simulink model "IMU_Uno"  (R2025b)
settings: Solver=FixedStepAuto  StartTime=0.0  StopTime=inf  FixedStep=Ts  RelTol=1e-3  EnableMultiTasking=on
InitFcn:
  | Ts=0.01;
  | Delay=5;
  | Av=50;
  | Sample_div=uint8(9);
  | Filter_BW=uint8(5);  %bandwidth 10 Hz
  | Gy_Conf=uint8(24); %-2000dps to 2000dps
  | Acc_Conf1=uint8(0); % -2g to 2g
  | Acc_Conf2=uint8(5); % bandwidth 10 Hz
  | FIFO_en=uint8(0); % Disabled
  | INT_en=uint8(0); % Disabled
  | Acc_Scale=9.8*2/32767;
  | Gyro_Scale=(2000*pi/180)/32767;
  | g_offset=16384;
  | 
  | %Registers
  | IMU_ID=113;
  | IMU_Add=104;
  | Who_Am_I=117;
  | PWR_1=107;
  | PWR_2=108;
  | SAMPL_DIV=25;
  | CONFIG_REG=26;
  | GYRO_CONFIG=27;
  | ACC_CONFIG_1=28;
  | ACC_CONFIG_2=29;
  | FIFO_EN=35;
  | INT_EN=56;
  | GY_X_OFFSET_H=19;
  | GY_X_OFFSET_L=20;
  | GY_Y_OFFSET_H=21;
  | GY_Y_OFFSET_L=22;
  | GY_Z_OFFSET_H=23;
  | GY_Z_OFFSET_L=24;
  | ACC_X_OFFSET_H=119;
  | ACC_X_OFFSET_L=120;
  | ACC_Y_OFFSET_H=122;
  | ACC_Y_OFFSET_L=123;
  | ACC_Z_OFFSET_H=125;
  | ACC_Z_OFFSET_L=126;
  | ACCEL_XOUT_H=59;
  | ACCEL_XOUT_L=60;
  | ACCEL_YOUT_H=61;
  | ACCEL_YOUT_L=62;
  | ACCEL_ZOUT_H=63;
  | ACCEL_ZOUT_L=64;
  | GYRO_XOUT_H=67;
  | GYRO_XOUT_L=68;
  | GYRO_YOUT_H=69;
  | GYRO_YOUT_L=70;
  | GYRO_ZOUT_H=71;
  | GYRO_ZOUT_L=72;
libraries: arduinolib x18
settings Model: SimulationMode=external  ExtModeTrigDuration=2  Creator=amind  LastModifiedBy=Amin Danial
settings SolverCC: AlgebraicLoopSolver=TrustRegion  AutoInsertRateTranBlk=on
settings DataIOCC: ReturnWorkspaceOutputs=off
settings OptimizationCC: EnhancedBackFolding=on  PassReuseOutputArgsAs=Individual arguments  MaxStackSize=64  OptimizeBlockOrder=speed  DifferentSizesBufferReuse=on  OptimizationCustomize=off  EfficientTunableParamExpr=on
settings DebuggingCC: ParameterPrecisionLossMsg=none  ParameterTunabilityLossMsg=error  UnconnectedInputMsg=warning  UnconnectedOutputMsg=warning  UnconnectedLineMsg=warning  ArithmeticOperatorsInVariantConditions=warning
settings HardwareCC: ProdBitPerInt=16.0  ProdBitPerPointer=16.0  ProdBitPerSizeT=16.0  ProdBitPerPtrDiffT=16.0  ProdLargestAtomicFloat=None  ProdWordSize=8.0  ProdHWDeviceType=Atmel->AVR
settings ModelReferenceCC: EnableRefExpFcnMdlSchedulingChecks=on
settings SFSimCC: MATLABDynamicMemAlloc=off  CustomCodeUndefinedFunction=UseInterfaceOnly
settings RTWCC: SystemTargetFile=ert.tlc  HardwareBoard=Arduino Uno  TemplateMakefile=ert_default_tmf  GenerateReport=on  Toolchain=Arduino AVR  BuildConfiguration=Faster Runs  IncludeHyperlinkInReport=on  LaunchReport=on  GenerateTraceInfo=on  GenerateTraceReport=on  GenerateTraceReportSl=on  GenerateTraceReportSf=on  GenerateTraceReportEml=on  GPUComputeCapability=3.5  Description=Embedded Coder
settings CodeAppCC: ForceParamTrailComments=on  IgnoreCustomStorageClasses=off  OperatorAnnotations=on  SimulinkDataObjDesc=on  SFDataObjDesc=on  InsertBlockDesc=on
settings ERTTargetCC: ExtModeTransport=3.0  ExtModeStaticAlloc=on  ExtModeAutomaticAllocSize=off  ExtModeStaticAllocSize=250.0  ExtModeMexFile=ext_xcp  ExtModeIntrfLevel=Level2 - Open  InlinedParameterPlacement=Hierarchical  DynamicArrayContainerType=coder::array  SupportContinuousTime=on  SupportVariableSizeSignals=on

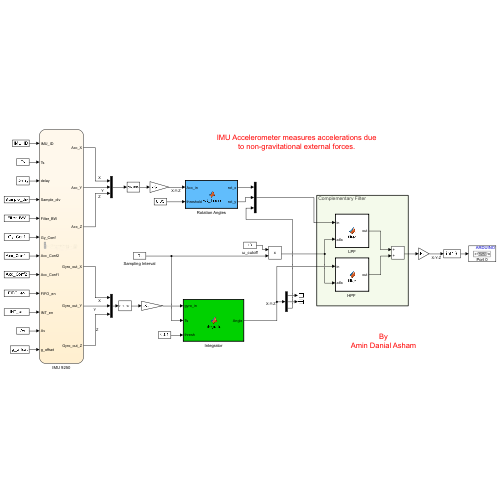
[thumbnail: Simulink's stored preview of the top-level diagram]
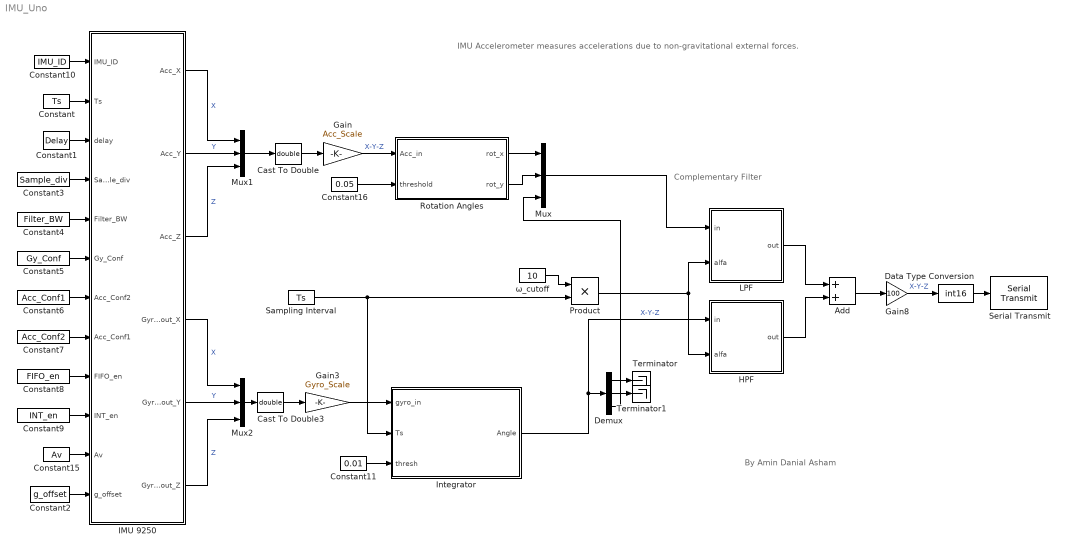
== system IMU_Uno ==
  note: By
      | Amin Danial Asham
  note: IMU Accelerometer measures accelerations due to non-gravitational external forces.
  note: Complementary Filter
  Add : Sum
  Cast To Double : DataTypeConversion  OutDataTypeStr=double  SaturateOnIntegerOverflow=off  RndMeth=Floor
  Cast To Double3 : DataTypeConversion  OutDataTypeStr=double  SaturateOnIntegerOverflow=off  RndMeth=Floor
  Constant : Constant  Value=Ts
  Constant1 : Constant  Value=Delay
  Constant10 : Constant  Value=IMU_ID
  Constant11 : Constant  Value=0.01
  Constant15 : Constant  Value=Av
  Constant16 : Constant  Value=0.05
  Constant2 : Constant  Value=g_offset
  Constant3 : Constant  Value=Sample_div
  Constant4 : Constant  Value=Filter_BW
  Constant5 : Constant  Value=Gy_Conf
  Constant6 : Constant  Value=Acc_Conf1
  Constant7 : Constant  Value=Acc_Conf2
  Constant8 : Constant  Value=FIFO_en
  Constant9 : Constant  Value=INT_en
  Data Type Conversion : DataTypeConversion  OutDataTypeStr=int16  SaturateOnIntegerOverflow=off  RndMeth=Floor
  Demux : Demux  Outputs=3
  Gain : Gain  Gain=Acc_Scale
  Gain3 : Gain  Gain=Gyro_Scale
  Gain8 : Gain  Gain=100
  "HPF " : MATLAB Function  TreatAsAtomicUnit=on
  IMU 9250 : Stateflow chart  TreatAsAtomicUnit=on  SystemSampleTime=Ts
  Integrator : MATLAB Function  InitFcn=|  TreatAsAtomicUnit=on
      | gyro=zeros(3,1);
      | gyro_1=zeros(3,1);
      | Angles=zeros(3,1);
  LPF : MATLAB Function  TreatAsAtomicUnit=on
  Mux : Mux  Inputs=3
  Mux1 : Mux  Inputs=3
  Mux2 : Mux  Inputs=3
  Product : Product
  Rotation Angles : MATLAB Function  TreatAsAtomicUnit=on
  Sampling Interval : Constant  Value=Ts
  Serial Transmit : arduinolib/Serial Transmit  portNumber=0  sendmode=write  sendformat=Decimal  floatprecision=2  header=[]  terminator=[]  blockPlatform=arduino
  Terminator : Terminator
  Terminator1 : Terminator
  ω_cutoff : Constant  Value=10
  wires:
  IMU 9250/1(Acc_X) -> Mux1/1  "X"
  IMU 9250/3(Acc_Z) -> Mux1/3  "Z"
  IMU 9250/2(Acc_Y) -> Mux1/2  "Y"
  Rotation Angles/1(rot_x) -> Mux/1
  Rotation Angles/2(rot_y) -> Mux/2
  Mux2/1 -> Cast To Double3/1
  IMU 9250/4(Gyro_out_X) -> Mux2/1  "X"
  IMU 9250/5(Gyro_out_Y) -> Mux2/2  "Y"
  IMU 9250/6(Gyro_out_Z) -> Mux2/3  "Z"
  Cast To Double3/1 -> Gain3/1
  Mux/1 -> LPF/1(in)
  Gain8/1 -> Data Type Conversion/1  "X-Y-Z"
  Data Type Conversion/1 -> Serial Transmit/1
  LPF/1(out) -> Add/1
  Mux1/1 -> Cast To Double/1
  Constant2/1 -> IMU 9250/12(g_offset)
  Constant15/1 -> IMU 9250/11(Av)
  Constant10/1 -> IMU 9250/1(IMU_ID)
  Constant6/1 -> IMU 9250/7(Acc_Conf2)
  Constant3/1 -> IMU 9250/4(Sample_div)
  Constant4/1 -> IMU 9250/5(Filter_BW)
  Constant5/1 -> IMU 9250/6(Gy_Conf)
  Constant9/1 -> IMU 9250/10(INT_en)
  Constant1/1 -> IMU 9250/3(delay)
  Constant7/1 -> IMU 9250/8(Acc_Conf1)
  Constant/1 -> IMU 9250/2(Ts)
  Constant8/1 -> IMU 9250/9(FIFO_en)
  Constant16/1 -> Rotation Angles/2(threshold)
  Cast To Double/1 -> Gain/1
  Gain/1 -> Rotation Angles/1(Acc_in)  "X-Y-Z"
  Product/1 -> LPF/2(alfa), "HPF "/2(alfa)
  Integrator/1(Angle) -> "HPF "/1(in), Demux/1  "X-Y-Z"
  Demux/3 -> Mux/3
  Demux/1 -> Terminator/1
  Demux/2 -> Terminator1/1
  "HPF "/1(out) -> Add/2
  Add/1 -> Gain8/1
  Sampling Interval/1 -> Integrator/2(Ts), Product/2
  ω_cutoff/1 -> Product/1
  Gain3/1 -> Integrator/1(gyro_in)
  Constant11/1 -> Integrator/3(thresh)

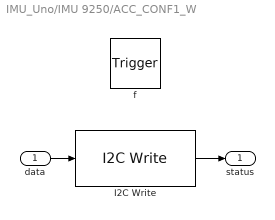
== system IMU_Uno/IMU 9250/ACC_CONF1_W ==
  data : Inport  OutDataTypeStr=uint8  PortDimensions=1
  f : TriggerPort  TriggerType=function-call  VariantControl=(inherit)
      settings: CopyFcn=Stateflow.SLINSF.SimulinkMan.removeBlockPreDeleteFcn  PreDeleteFcn=Stateflow.SLINSF.SimulinkMan.unsafePredeleteFcn
  I2C Write : arduinolib/I2C Write  I2CModule=0  Mode=Master  SlaveAddress=IMU_Add  SlaveByteOrder=BigEndian  Direction=Transmitter  RegisterAddressMode=on  RegisterAddress=ACC_CONFIG_1  SlaveDataType=uint8  DataLength=1  NoAck=off  RepeatedStart=off  OutputStatus=on  blockPlatform=ARDUINO
  status : Outport  VectorParamsAs1DForOutWhenUnconnected=off
  wires:
  I2C Write/1 -> status/1
  data/1 -> I2C Write/1

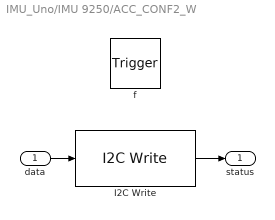
== system IMU_Uno/IMU 9250/ACC_CONF2_W ==
  data : Inport  OutDataTypeStr=uint8  PortDimensions=1
  f : TriggerPort  TriggerType=function-call  VariantControl=(inherit)
      settings: CopyFcn=Stateflow.SLINSF.SimulinkMan.removeBlockPreDeleteFcn  PreDeleteFcn=Stateflow.SLINSF.SimulinkMan.unsafePredeleteFcn
  I2C Write : arduinolib/I2C Write  I2CModule=0  Mode=Master  SlaveAddress=IMU_Add  SlaveByteOrder=BigEndian  Direction=Transmitter  RegisterAddressMode=on  RegisterAddress=ACC_CONFIG_2  SlaveDataType=uint8  DataLength=1  NoAck=off  RepeatedStart=off  OutputStatus=on  blockPlatform=ARDUINO
  status : Outport  VectorParamsAs1DForOutWhenUnconnected=off
  wires:
  I2C Write/1 -> status/1
  data/1 -> I2C Write/1

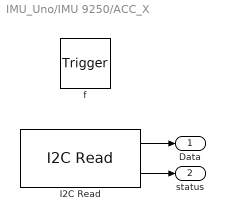
== system IMU_Uno/IMU 9250/ACC_X ==
  f : TriggerPort  TriggerType=function-call  VariantControl=(inherit)
      settings: CopyFcn=Stateflow.SLINSF.SimulinkMan.removeBlockPreDeleteFcn  PreDeleteFcn=Stateflow.SLINSF.SimulinkMan.unsafePredeleteFcn
  I2C Read : arduinolib/I2C Read  I2CModule=0  Mode=Master  SlaveAddress=IMU_Add  SlaveByteOrder=BigEndian  Direction=Receiver  RegisterAddressMode=on  RegisterAddress=ACCEL_XOUT_H  SlaveDataType=int16  DataLength=1  NoAck=off  RepeatedStart=off  OutputStatus=on  blockPlatform=ARDUINO  SampleTime=-1
  Data : Outport  VectorParamsAs1DForOutWhenUnconnected=off
  status : Outport  Port=2  VectorParamsAs1DForOutWhenUnconnected=off
  wires:
  I2C Read/1 -> Data/1
  I2C Read/2 -> status/1

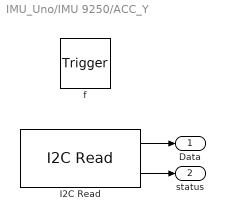
== system IMU_Uno/IMU 9250/ACC_Y ==
  f : TriggerPort  TriggerType=function-call  VariantControl=(inherit)
      settings: CopyFcn=Stateflow.SLINSF.SimulinkMan.removeBlockPreDeleteFcn  PreDeleteFcn=Stateflow.SLINSF.SimulinkMan.unsafePredeleteFcn
  I2C Read : arduinolib/I2C Read  I2CModule=0  Mode=Master  SlaveAddress=IMU_Add  SlaveByteOrder=BigEndian  Direction=Receiver  RegisterAddressMode=on  RegisterAddress=ACCEL_YOUT_H  SlaveDataType=int16  DataLength=1  NoAck=off  RepeatedStart=off  OutputStatus=on  blockPlatform=ARDUINO  SampleTime=-1
  Data : Outport  VectorParamsAs1DForOutWhenUnconnected=off
  status : Outport  Port=2  VectorParamsAs1DForOutWhenUnconnected=off
  wires:
  I2C Read/1 -> Data/1
  I2C Read/2 -> status/1

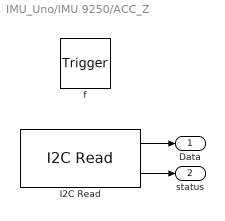
== system IMU_Uno/IMU 9250/ACC_Z ==
  f : TriggerPort  TriggerType=function-call  VariantControl=(inherit)
      settings: CopyFcn=Stateflow.SLINSF.SimulinkMan.removeBlockPreDeleteFcn  PreDeleteFcn=Stateflow.SLINSF.SimulinkMan.unsafePredeleteFcn
  I2C Read : arduinolib/I2C Read  I2CModule=0  Mode=Master  SlaveAddress=IMU_Add  SlaveByteOrder=BigEndian  Direction=Receiver  RegisterAddressMode=on  RegisterAddress=ACCEL_ZOUT_H  SlaveDataType=int16  DataLength=1  NoAck=off  RepeatedStart=off  OutputStatus=on  blockPlatform=ARDUINO  SampleTime=-1
  Data : Outport  VectorParamsAs1DForOutWhenUnconnected=off
  status : Outport  Port=2  VectorParamsAs1DForOutWhenUnconnected=off
  wires:
  I2C Read/1 -> Data/1
  I2C Read/2 -> status/1

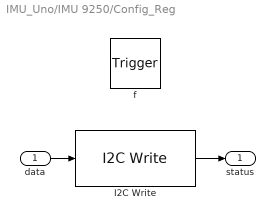
== system IMU_Uno/IMU 9250/Config_Reg ==
  data : Inport  OutDataTypeStr=uint8  PortDimensions=1
  f : TriggerPort  TriggerType=function-call  VariantControl=(inherit)
      settings: CopyFcn=Stateflow.SLINSF.SimulinkMan.removeBlockPreDeleteFcn  PreDeleteFcn=Stateflow.SLINSF.SimulinkMan.unsafePredeleteFcn
  I2C Write : arduinolib/I2C Write  I2CModule=0  Mode=Master  SlaveAddress=IMU_Add  SlaveByteOrder=BigEndian  Direction=Transmitter  RegisterAddressMode=on  RegisterAddress=CONFIG_REG  SlaveDataType=uint8  DataLength=1  NoAck=off  RepeatedStart=off  OutputStatus=on  blockPlatform=ARDUINO
  status : Outport  VectorParamsAs1DForOutWhenUnconnected=off
  wires:
  I2C Write/1 -> status/1
  data/1 -> I2C Write/1

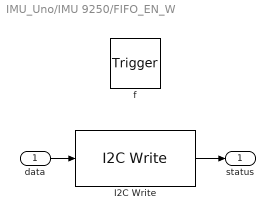
== system IMU_Uno/IMU 9250/FIFO_EN_W ==
  data : Inport  OutDataTypeStr=uint8  PortDimensions=1
  f : TriggerPort  TriggerType=function-call  VariantControl=(inherit)
      settings: CopyFcn=Stateflow.SLINSF.SimulinkMan.removeBlockPreDeleteFcn  PreDeleteFcn=Stateflow.SLINSF.SimulinkMan.unsafePredeleteFcn
  I2C Write : arduinolib/I2C Write  I2CModule=0  Mode=Master  SlaveAddress=IMU_Add  SlaveByteOrder=BigEndian  Direction=Transmitter  RegisterAddressMode=on  RegisterAddress=FIFO_EN  SlaveDataType=uint8  DataLength=1  NoAck=off  RepeatedStart=off  OutputStatus=on  blockPlatform=ARDUINO
  status : Outport  VectorParamsAs1DForOutWhenUnconnected=off
  wires:
  I2C Write/1 -> status/1
  data/1 -> I2C Write/1

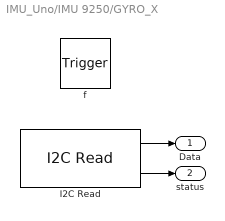
== system IMU_Uno/IMU 9250/GYRO_X ==
  f : TriggerPort  TriggerType=function-call  VariantControl=(inherit)
      settings: CopyFcn=Stateflow.SLINSF.SimulinkMan.removeBlockPreDeleteFcn  PreDeleteFcn=Stateflow.SLINSF.SimulinkMan.unsafePredeleteFcn
  I2C Read : arduinolib/I2C Read  I2CModule=0  Mode=Master  SlaveAddress=IMU_Add  SlaveByteOrder=BigEndian  Direction=Receiver  RegisterAddressMode=on  RegisterAddress=GYRO_XOUT_H  SlaveDataType=int16  DataLength=1  NoAck=off  RepeatedStart=off  OutputStatus=on  blockPlatform=ARDUINO  SampleTime=-1
  Data : Outport  VectorParamsAs1DForOutWhenUnconnected=off
  status : Outport  Port=2  VectorParamsAs1DForOutWhenUnconnected=off
  wires:
  I2C Read/1 -> Data/1
  I2C Read/2 -> status/1

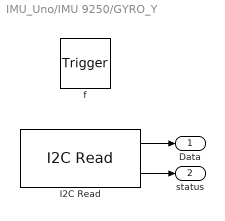
== system IMU_Uno/IMU 9250/GYRO_Y ==
  f : TriggerPort  TriggerType=function-call  VariantControl=(inherit)
      settings: CopyFcn=Stateflow.SLINSF.SimulinkMan.removeBlockPreDeleteFcn  PreDeleteFcn=Stateflow.SLINSF.SimulinkMan.unsafePredeleteFcn
  I2C Read : arduinolib/I2C Read  I2CModule=0  Mode=Master  SlaveAddress=IMU_Add  SlaveByteOrder=BigEndian  Direction=Receiver  RegisterAddressMode=on  RegisterAddress=GYRO_YOUT_H  SlaveDataType=int16  DataLength=1  NoAck=off  RepeatedStart=off  OutputStatus=on  blockPlatform=ARDUINO  SampleTime=-1
  Data : Outport  VectorParamsAs1DForOutWhenUnconnected=off
  status : Outport  Port=2  VectorParamsAs1DForOutWhenUnconnected=off
  wires:
  I2C Read/1 -> Data/1
  I2C Read/2 -> status/1

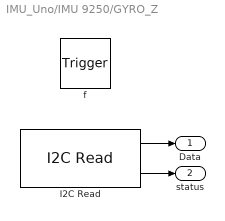
== system IMU_Uno/IMU 9250/GYRO_Z ==
  f : TriggerPort  TriggerType=function-call  VariantControl=(inherit)
      settings: CopyFcn=Stateflow.SLINSF.SimulinkMan.removeBlockPreDeleteFcn  PreDeleteFcn=Stateflow.SLINSF.SimulinkMan.unsafePredeleteFcn
  I2C Read : arduinolib/I2C Read  I2CModule=0  Mode=Master  SlaveAddress=IMU_Add  SlaveByteOrder=BigEndian  Direction=Receiver  RegisterAddressMode=on  RegisterAddress=GYRO_ZOUT_H  SlaveDataType=int16  DataLength=1  NoAck=off  RepeatedStart=off  OutputStatus=on  blockPlatform=ARDUINO  SampleTime=-1
  Data : Outport  VectorParamsAs1DForOutWhenUnconnected=off
  status : Outport  Port=2  VectorParamsAs1DForOutWhenUnconnected=off
  wires:
  I2C Read/1 -> Data/1
  I2C Read/2 -> status/1

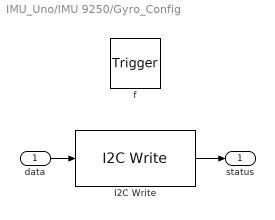
== system IMU_Uno/IMU 9250/Gyro_Config ==
  data : Inport  OutDataTypeStr=uint8  PortDimensions=1
  f : TriggerPort  TriggerType=function-call  VariantControl=(inherit)
      settings: CopyFcn=Stateflow.SLINSF.SimulinkMan.removeBlockPreDeleteFcn  PreDeleteFcn=Stateflow.SLINSF.SimulinkMan.unsafePredeleteFcn
  I2C Write : arduinolib/I2C Write  I2CModule=0  Mode=Master  SlaveAddress=IMU_Add  SlaveByteOrder=BigEndian  Direction=Transmitter  RegisterAddressMode=on  RegisterAddress=GYRO_CONFIG  SlaveDataType=uint8  DataLength=1  NoAck=off  RepeatedStart=off  OutputStatus=on  blockPlatform=ARDUINO
  status : Outport  VectorParamsAs1DForOutWhenUnconnected=off
  wires:
  I2C Write/1 -> status/1
  data/1 -> I2C Write/1

== system IMU_Uno/IMU 9250/INT_EN_W ==
  data : Inport  OutDataTypeStr=uint8  PortDimensions=1
  f : TriggerPort  TriggerType=function-call  VariantControl=(inherit)
      settings: CopyFcn=Stateflow.SLINSF.SimulinkMan.removeBlockPreDeleteFcn  PreDeleteFcn=Stateflow.SLINSF.SimulinkMan.unsafePredeleteFcn
  I2C Write : arduinolib/I2C Write  I2CModule=0  Mode=Master  SlaveAddress=IMU_Add  SlaveByteOrder=BigEndian  Direction=Transmitter  RegisterAddressMode=on  RegisterAddress=INT_EN  SlaveDataType=uint8  DataLength=1  NoAck=off  RepeatedStart=off  OutputStatus=on  blockPlatform=ARDUINO
  status : Outport  VectorParamsAs1DForOutWhenUnconnected=off
  wires:
  I2C Write/1 -> status/1
  data/1 -> I2C Write/1

== system IMU_Uno/IMU 9250/PWR1_R ==
  f : TriggerPort  TriggerType=function-call  VariantControl=(inherit)
      settings: CopyFcn=Stateflow.SLINSF.SimulinkMan.removeBlockPreDeleteFcn  PreDeleteFcn=Stateflow.SLINSF.SimulinkMan.unsafePredeleteFcn
  PWR 1 : arduinolib/I2C Read  I2CModule=0  Mode=Master  SlaveAddress=IMU_Add  SlaveByteOrder=BigEndian  Direction=Receiver  RegisterAddressMode=on  RegisterAddress=PWR_1  SlaveDataType=uint8  DataLength=1  NoAck=off  RepeatedStart=off  OutputStatus=on  blockPlatform=ARDUINO  SampleTime=-1
  data : Outport  VectorParamsAs1DForOutWhenUnconnected=off
  status : Outport  Port=2  VectorParamsAs1DForOutWhenUnconnected=off
  wires:
  PWR 1/1 -> data/1
  PWR 1/2 -> status/1

== system IMU_Uno/IMU 9250/PWR1_W ==
  data : Inport  OutDataTypeStr=uint8  PortDimensions=1
  f : TriggerPort  TriggerType=function-call  VariantControl=(inherit)
      settings: CopyFcn=Stateflow.SLINSF.SimulinkMan.removeBlockPreDeleteFcn  PreDeleteFcn=Stateflow.SLINSF.SimulinkMan.unsafePredeleteFcn
  PWR 1 1 : arduinolib/I2C Write  I2CModule=0  Mode=Master  SlaveAddress=IMU_Add  SlaveByteOrder=BigEndian  Direction=Transmitter  RegisterAddressMode=on  RegisterAddress=PWR_1  SlaveDataType=uint8  DataLength=1  NoAck=off  RepeatedStart=off  OutputStatus=on  blockPlatform=ARDUINO
  status : Outport  VectorParamsAs1DForOutWhenUnconnected=off
  wires:
  data/1 -> PWR 1 1/1
  PWR 1 1/1 -> status/1

== system IMU_Uno/IMU 9250/PWR2_W ==
  data : Inport  OutDataTypeStr=uint8  PortDimensions=1
  f : TriggerPort  TriggerType=function-call  VariantControl=(inherit)
      settings: CopyFcn=Stateflow.SLINSF.SimulinkMan.removeBlockPreDeleteFcn  PreDeleteFcn=Stateflow.SLINSF.SimulinkMan.unsafePredeleteFcn
  I2C Write : arduinolib/I2C Write  I2CModule=0  Mode=Master  SlaveAddress=IMU_Add  SlaveByteOrder=BigEndian  Direction=Transmitter  RegisterAddressMode=on  RegisterAddress=PWR_2  SlaveDataType=uint8  DataLength=1  NoAck=off  RepeatedStart=off  OutputStatus=on  blockPlatform=ARDUINO
  status : Outport  VectorParamsAs1DForOutWhenUnconnected=off
  wires:
  data/1 -> I2C Write/1
  I2C Write/1 -> status/1

== system IMU_Uno/IMU 9250/SAMPL_Div ==
  data : Inport  OutDataTypeStr=uint8  PortDimensions=1
  f : TriggerPort  TriggerType=function-call  VariantControl=(inherit)
      settings: CopyFcn=Stateflow.SLINSF.SimulinkMan.removeBlockPreDeleteFcn  PreDeleteFcn=Stateflow.SLINSF.SimulinkMan.unsafePredeleteFcn
  I2C Write : arduinolib/I2C Write  I2CModule=0  Mode=Master  SlaveAddress=IMU_Add  SlaveByteOrder=BigEndian  Direction=Transmitter  RegisterAddressMode=on  RegisterAddress=SAMPL_DIV  SlaveDataType=uint8  DataLength=1  NoAck=off  RepeatedStart=off  OutputStatus=on  blockPlatform=ARDUINO
  status : Outport  VectorParamsAs1DForOutWhenUnconnected=off
  wires:
  I2C Write/1 -> status/1
  data/1 -> I2C Write/1

== system IMU_Uno/IMU 9250/Stop ==
  f : TriggerPort  TriggerType=function-call  VariantControl=(inherit)
      settings: CopyFcn=Stateflow.SLINSF.SimulinkMan.removeBlockPreDeleteFcn  PreDeleteFcn=Stateflow.SLINSF.SimulinkMan.unsafePredeleteFcn
  Constant : Constant
  Stop Simulation : Stop
  wires:
  Constant/1 -> Stop Simulation/1

== system IMU_Uno/IMU 9250/Who_Am_I ==
  f : TriggerPort  TriggerType=function-call  VariantControl=(inherit)
      settings: CopyFcn=Stateflow.SLINSF.SimulinkMan.removeBlockPreDeleteFcn  PreDeleteFcn=Stateflow.SLINSF.SimulinkMan.unsafePredeleteFcn
  I2C Read : arduinolib/I2C Read  I2CModule=0  Mode=Master  SlaveAddress=IMU_Add  SlaveByteOrder=BigEndian  Direction=Receiver  RegisterAddressMode=on  RegisterAddress=Who_Am_I  SlaveDataType=uint8  DataLength=1  NoAck=off  RepeatedStart=off  OutputStatus=on  blockPlatform=ARDUINO  SampleTime=-1
  data : Outport  VectorParamsAs1DForOutWhenUnconnected=off
  status : Outport  Port=2  VectorParamsAs1DForOutWhenUnconnected=off
  wires:
  I2C Read/2 -> status/1
  I2C Read/1 -> data/1

== matlab function IMU_Uno/Rotation Angles ==
  data: Acc_in input; rot_x output; rot_y output; threshold input
function [rot_x,rot_y] = Rot_Trans(Acc_in,threshold)
% The order of rotation z,y,x of the IMU
  x=Acc_in(1);
  y=Acc_in(2);
  z=Acc_in(3);
  if(abs(x)<=threshold)
      x=0;
  end
  if(abs(y)<=threshold)
      y=0;
  end
  if(abs(z)<=threshold)
      z=0;
  end
  rot_x=atan2(y,z);
  rot_y=atan2(-x,sqrt(y^2+z^2));
  end

== stateflow chart IMU_Uno/IMU 9250 ==
  state Stop [function]
  state [data,status] = Who_Am_I [function]
  state [data,status] = PWR1_R [function]
  state status=PWR1_W(data) [function]
  state status=PWR2_W(data) [function]
  state status = SAMPL_Div(data) [function]
  state status = Config_Reg(data) [function]
  state Measurments
    en:
    status=uint8(1);
    status1=uint8(1);
    status2=uint8(1);
    status3=uint8(1);
    status4=uint8(1);
    status5=uint8(1);
    state ACC_X
      du:
      [temp,status] = ACC_X;
      Acc_X=temp-acc_offset_x;
    state ACC_Y
      du:
      [ temp,status1] = ACC_Y;
      Acc_Y=temp-acc_offset_y;
    state ACC_Z
      du:
      [temp,status2] = ACC_Z;
      Acc_Z=temp-acc_offset_z+g_offset;
    state GYRO_X
      du:
      [temp,status3] = GYRO_X;
      Gyro_out_X=temp-gyro_offset_x
    state GYRO_Y
      du:
      [temp,status4] = GYRO_Y;
      Gyro_out_Y=temp-gyro_offset_y
    state GYRO_Z
      du:
      [temp,status5] = GYRO_Z;
      Gyro_out_Z=temp-gyro_offset_z
    (default) -> ACC_X
    ACC_X -> ACC_Y : [status==0]
    ACC_Y -> ACC_Z : [status1==0]
    ACC_Z -> GYRO_X : [status2==0]
    GYRO_X -> GYRO_Y : [status3==0]
    GYRO_Y -> GYRO_Z : [status4==0]
  state Calibration
    en:
    status=uint8(1);
    status1=uint8(1);
    status2=uint8(1);
    status3=uint8(1);
    status4=uint8(1);
    status5=uint8(1);;
    state ACC_OFFSET_X
      du:
      [temp,status] = ACC_X;
      acc_offset_x=acc_offset_x+double(temp);
    state ACC_OFFSET_Y
      du:
      [temp,status1] = ACC_Y;
      acc_offset_y=acc_offset_y+double(temp);
    state ACC_OFFSET_Z
      du:
      [temp,status2] = ACC_Z;
      acc_offset_z=acc_offset_z+double(temp);
    state GYRO_OFFSET_X
      du:
      [temp,status3] = GYRO_X;
      gyro_offset_x=gyro_offset_x+double(temp);
    state GYRO_OFFSET_Y
      du:
      [ temp,status4] = GYRO_Y;
      gyro_offset_y=gyro_offset_y+double(temp);
    state GYRO_OFFSET_Z
      du:
      [temp,status5] = GYRO_Z;
      gyro_offset_z=gyro_offset_z+double(temp);
    (default) -> ACC_OFFSET_X
    ACC_OFFSET_X -> ACC_OFFSET_Y : [status==0]
    ACC_OFFSET_Y -> ACC_OFFSET_Z : [status1==0]
    ACC_OFFSET_Z -> GYRO_OFFSET_X : [status2==0]
    GYRO_OFFSET_X -> GYRO_OFFSET_Y : [status3==0]
    GYRO_OFFSET_Y -> GYRO_OFFSET_Z : [status4==0]
  state PWR_Adj
    en:
    status=uint8(1);
    status1=uint8(1);
    status2=uint8(1);
    state PWR1_R
      du:
      [data,status]=PWR1_R();
    state PWR1_W
      du:
      status1=PWR1_W(uint8(and(5,data)));
    state PWR2_W1
      du:
      status2= PWR2_W(uint8(0));
    (default) -> PWR1_R
    PWR1_R -> PWR1_W : [status==0]
    PWR1_W -> PWR2_W1 : [status1==0]
  state status = Gyro_Config(data) [function]
  state Acc_Conf
    en:
    status=uint8(1);
    status1=uint8(1);
    state ACC_Conf1
      du:
      status = ACC_CONF1_W(Acc_Conf1);
    state ACC_Conf2
      du:
      status1 = ACC_CONF2_W(Acc_Conf2);
    (default) -> ACC_Conf1
    ACC_Conf1 -> ACC_Conf2 : [status==0]
  state status = ACC_CONF1_W(data) [function]
  state status = ACC_CONF2_W(data) [function]
  state INT
    en:
    status=uint8(1);
    du:
    status=INT_EN_W(INT_en);
  state FIFO
    en:
    status=uint8(1);
    du:
    status=FIFO_EN_W(FIFO_en);
  state SAMPL_Rate_Div
    en:
    status=uint8(1);
    du:
    status=SAMPL_Div(Sample_div);
  state Config
    en:
    status=uint8(1);
    du:
    status = Config_Reg(Filter_BW);
  state Gyro_Conf
    en:
    status=uint8(1);
    du:
    status=Gyro_Config(Gy_Conf);
  state Identification
    en:
    status=uint8(1);
    data=uint8(0);
    du:
    [data,status]=Who_Am_I();
    ID=data;
  state status = FIFO_EN_W(data) [function]
  state status = INT_EN_W(data) [function]
  state [Data,status] = ACC_X [function]
  state [Data,status] = ACC_Y [function]
  state [Data,status] = ACC_Z [function]
  state [Data,status] = GYRO_X [function]
  state Stopping
    en:
    Error=status;
    Stop();
  state [Data,status] = GYRO_Y [function]
  state [Data,status] = GYRO_Z [function]
  PWR_Adj -> SAMPL_Rate_Div [order 2] : [status==0 && status1==0 && status2==0]
  Acc_Conf -> FIFO [order 2] : [status==0 && status1==0]
  Calibration -> Measurments [order 1] : [status==0 && status1==0 && status2==0 && status3==0 && status4==0 && status5==0 && cnt==Av]
      | {acc_offset_x=acc_offset_x/cnt;
      | acc_offset_y=acc_offset_y/cnt;
      | acc_offset_z=acc_offset_z/cnt;
      | gyro_offset_x=gyro_offset_x/cnt;
      | gyro_offset_y=gyro_offset_y/cnt;
      | gyro_offset_z=gyro_offset_z/cnt;}
  (default) -> Identification
  FIFO -> INT [order 2] : [status==0]
  SAMPL_Rate_Div -> Config [order 2] : [status==0]
  INT -> Calibration [order 1] : [status==0]{cnt=0;
      | acc_offset_x=0;
      | acc_offset_y=0;
      | acc_offset_z=0;
      | gyro_offset_x=0;
      | gyro_offset_y=0;
      | gyro_offset_z=0;
      | }
  Config -> Gyro_Conf [order 2] : [status==0]
  Gyro_Conf -> Acc_Conf [order 2] : [status==0]
  Identification -> PWR_Adj [order 1] : [status==0 && data==IMU_ID]
  SAMPL_Rate_Div -> Stopping [order 1] : after(delay,sec)
  FIFO -> Stopping [order 1] : after(delay,sec)
  INT -> Stopping [order 2] : after(delay,sec)
  Measurments -> (junction 253) [order 1] : [status==0 && status1==0 && status2==0 && status3==0 && status4==0 && status5==0]
  Config -> Stopping [order 1] : after(delay,sec)
  Gyro_Conf -> Stopping [order 1] : after(delay,sec)
  (junction 253) -> Measurments : after(Ts,sec)
  Calibration -> (junction 225) [order 3] : [status==0 && status1==0 && status2==0 && status3==0 && status4==0 && status5==0]
      | {cnt=cnt+1;}
  (junction 225) -> Calibration : after(Ts,sec)
  Identification -> Stopping [order 2] : after(delay,sec)
  Acc_Conf -> Stopping [order 1] : after(delay,sec)
  PWR_Adj -> Stopping [order 1] : after(delay,sec)
  Calibration -> Stopping [order 2] : after(delay,sec)
  Measurments -> Stopping [order 2] : after(delay,sec)
  data: data function_output; status function_output; data function_output; status function_output; data function_input uint8 size=1; status function_output; data function_input uint8 size=1; status function_output; data function_input uint8 size=1; status function_output; data function_input uint8 size=1; status function_output; data function_input uint8 size=1; status function_output; data function_input uint8 size=1; status function_output; data function_input uint8 size=1; status function_output; data function_input uint8 size=1; status function_output; data function_input uint8 size=1; status function_output; Data function_output; status function_output; Data function_output; status function_output; Data function_output; status function_output; Data function_output; status function_output; Data function_output; status function_output; Data function_output; status function_output; IMU_ID input; data local; status local; Acc_X output; Acc_Y output; Ts input; delay input; Sample_div input; Filter_BW input; Gy_Conf input; Acc_Conf2 input; Acc_Conf1 input; FIFO_en input; INT_en input; Acc_Z output; Gyro_out_X output; scale local; temp local; status2 local; status1 local; Av input; Gyro_out_Y output; Gyro_out_Z output; status4 local; status5 local; status3 local; gyro_offset_x local; gyro_offset_y local; gyro_offset_z local; g_offset input; acc_offset_y local; acc_offset_x local; acc_offset_z local; Error local; ID local; cnt local

== matlab function IMU_Uno/Integrator ==
  data: gyro_in input; Angle output; Ts input; thresh input
function Angle = Integrator(gyro_in,Ts,thresh)
    persistent gyro_1 angle
    if isempty(gyro_1)
        gyro_1=zeros(3,1);
        angle=zeros(3,1);
    end
    x=gyro_in(1);
    y=gyro_in(2);
    z=gyro_in(3);
    if(abs(x)<=thresh)
      x=0;
    end
    if(abs(y)<=thresh)
      y=0;
    end
    if(abs(z)<=thresh)
      z=0;
    end
    gyro=[x;y;z];
    angle = angle+(gyro+gyro_1)*Ts/2;
    Angle=angle;
    gyro_1=gyro;
end

== matlab function IMU_Uno/LPF ==
  data: in input; out output; alfa input
function out = filter(in,alfa)
   persistent out_1
   if isempty(out_1)
       out_1=zeros(3,1);
   end
   out=in*alfa/(alfa+1)+out_1/(alfa+1);
   out_1=out;
end

== matlab function IMU_Uno/HPF  ==
  data: in input; out output; alfa input
function out = filter(in,alfa)
    persistent out_1 in_1
    if isempty(out_1)
        out_1=zeros(3,1);
        in_1=zeros(3,1);
    end
    out=(in-in_1+out_1)/(alfa+1);
    out_1=out;
    in_1=in;
end
